simulink model "Bus_creator_and_scope"  (R2016a)
settings: Solver=VariableStepAuto  StartTime=0.0  StopTime=10.0  RelTol=1e-3
settings Model: Creator=33105  LastModifiedBy=33105

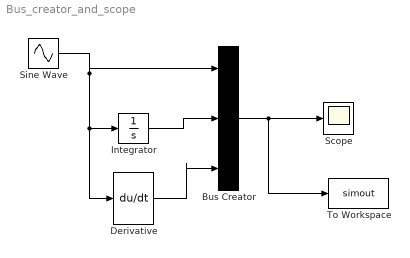
== system Bus_creator_and_scope ==
  Bus Creator : BusCreator  Inputs=3
  Derivative : Derivative
  Integrator : Integrator
  Scope : Scope
  Sine Wave : Sin  SampleTime=0
  To Workspace : ToWorkspace  VariableName=simout  SaveFormat=Timeseries  SampleTime=-1
  wires:
  Sine Wave/1 -> Bus Creator/1, Derivative/1, Integrator/1
  Integrator/1 -> Bus Creator/2
  Derivative/1 -> Bus Creator/3
  Bus Creator/1 -> To Workspace/1, Scope/1
